simulink model "B1_quadcopter_model"  (R2021b)
settings: Solver=VariableStepAuto  StartTime=0.0  StopTime=10  RelTol=1e-3
values from neighbouring files (symbols this model uses):
  K_act = 50    [A10_simple_plant.m]    (also in A11_setup_script_pprz.m = 20; A1_setup_script.m = 20)
  K_act_inner = K_act*eye(4)    [A11_setup_script_pprz.m]    (also in A1_setup_script.m)
  K_u_d = 2.5    [A11_setup_script_pprz.m]    (also in A1_setup_script.m = 7)
  K_v_d = 2.5    [A11_setup_script_pprz.m]    (also in A1_setup_script.m = 7)
  K_w_d = 2.5    [A11_setup_script_pprz.m]    (also in A1_setup_script.m = 7)
  max_motor_rate = 30000    [A11_setup_script_pprz.m]    (also in A1_setup_script.m)
  max_omega_motor = 11000    [A11_setup_script_pprz.m]    (also in A1_setup_script.m)
  omega_c_motors = 50    [A11_setup_script_pprz.m]    (also in A1_setup_script.m)
  sampling_time = 1/frequency    (= 0.002)    [A11_setup_script_pprz.m]    (also in A12_sim_multi_run.m; A1_setup_script.m; A6_slow_actuator.m)
undefined symbols (not defined in the file or in its folder): K_ec_d_p, K_ec_d_q, K_ec_d_r, K_ec_dd_p, K_ec_dd_q, K_ec_dd_r, K_ec_p, K_ec_q, K_ec_r, K_p, K_p_d, K_p_dd, K_q, K_q_d, K_q_dd, K_r, K_r_d, K_r_dd
libraries: dspinverses x11, simulink_extras x6, sim3dlib x1, uavsim3dlib x1, vrlib x1, aerolibutil x1, sharedutil x1, aerolibbdyn x1, aerolibatmos2 x1
(part 2 of 3)

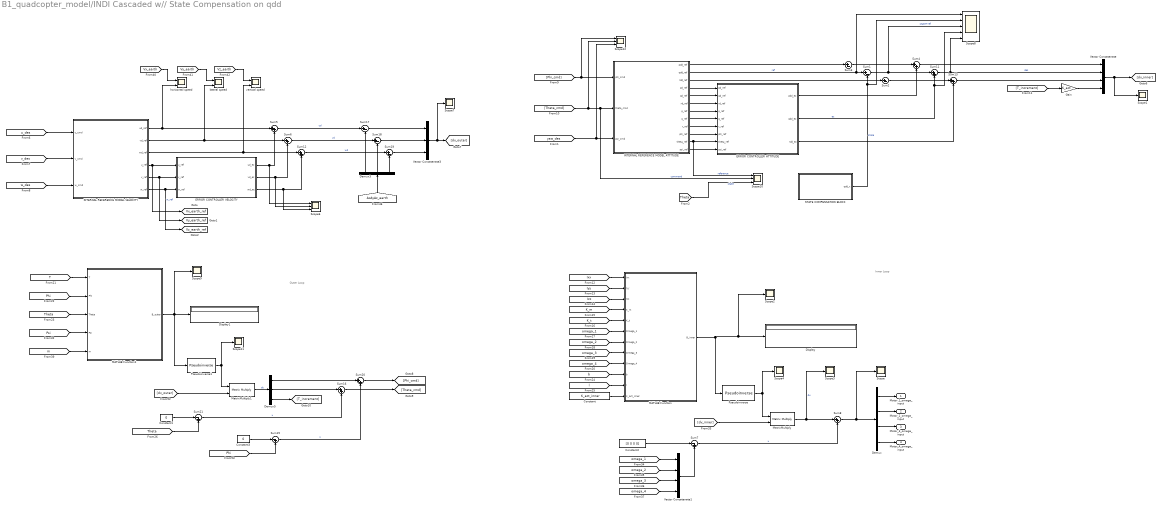
== system B1_quadcopter_model/INDI Cascaded w// State Compensation on qdd ==
  note: Outer Loop
  note: Inner Loop
  Constant : Constant  Value=K_act_inner
  Constant1 : Constant  Value=0
  Constant2 : Constant  Value=[0 0 0 0]
  Constant3 : Constant  Value=0
  Demux : Demux
  Demux3 : Demux  Outputs=3
  Demux5 : Demux  Outputs=3
  Display : Display
  Display1 : Display
  ERROR CONTROLLER ATTITUDE : Subsystem
  ERROR CONTROLLER VELOCITY : Subsystem
  Gain : Gain  Gain=K_act
  INTERNAL REFERENCE MODEL ATTITUDE : Subsystem
  INTERNAL REFERENCE MODEL VELOCITY : Subsystem
  MATLAB Function : MATLAB Function  TreatAsAtomicUnit=on
  MATLAB Function1 : MATLAB Function  TreatAsAtomicUnit=on
  MatrixMultiply : Product  Multiplication=Matrix(*)
  MatrixMultiply1 : Product  Multiplication=Matrix(*)
  Pseudoinverse : dspinverses/Pseudoinverse  wanterr=off  SimulateUsing=Interpreted execution
      settings: SourceProductBaseCode=DS
  Pseudoinverse1 : dspinverses/Pseudoinverse  wanterr=off  SimulateUsing=Interpreted execution
      settings: SourceProductBaseCode=DS
  STATE COMPENSATION BLOCK : Subsystem
  Scope{,1..4,7,9,11} (8 alike) : Scope
  Scope10 : Scope  NumInputPorts=3
  Scope12 : Scope  NumInputPorts=3
  Scope6 : Scope  NumInputPorts=3
  Scope8 : Scope  NumInputPorts=5
  Sum{1..3,17..19} (6 alike) : Sum  Inputs=|+-
  Sum{4..6,8,11..13,16,20} (9 alike) : Sum  Inputs=|++
  Sum15 : Sum  Inputs=|-+
  Sum21 : Sum  Inputs=|-+
  Sum7 : Sum  Inputs=|-+
  Vector Concatenate : Concatenate  NumInputs=4
  Vector Concatenate1 : Concatenate  NumInputs=4
  Vector Concatenate3 : Concatenate  NumInputs=3
  horizontal speed : Scope  NumInputPorts=2
  lateral speed : Scope  NumInputPorts=2
  vertical speed : Scope  NumInputPorts=2
  Motor_1_omega_input : Outport
  Motor_2_omega_input : Outport  Port=2
  Motor_3_omega_input : Outport  Port=3
  Motor_4_omega_input : Outport  Port=4
  tag scope: Vx_earth_ref=global, Vy_earth_ref=global, Vz_earth_ref=global
  wires:
  ERROR CONTROLLER VELOCITY/1(ud_ec) -> Sum5/2, Scope6/1
  ERROR CONTROLLER VELOCITY/3(wd_ec) -> Sum12/2, Scope6/3
  INTERNAL REFERENCE MODEL VELOCITY/3(wd_ref) -> vertical speed/2, Sum12/1
  INTERNAL REFERENCE MODEL VELOCITY/2(vd_ref) -> lateral speed/2, Sum6/1
  INTERNAL REFERENCE MODEL VELOCITY/5(v_ref) -> [Vy_earth_ref], ERROR CONTROLLER VELOCITY/2(v_ref)
  INTERNAL REFERENCE MODEL VELOCITY/6(w_ref) -> [Vz_earth_ref], ERROR CONTROLLER VELOCITY/3(w_ref)  "w_ref"
  INTERNAL REFERENCE MODEL VELOCITY/1(ud_ref) -> horizontal speed/2, Sum5/1
  ERROR CONTROLLER VELOCITY/2(vd_ec) -> Sum6/2, Scope6/2
  INTERNAL REFERENCE MODEL VELOCITY/4(u_ref) -> [Vx_earth_ref], ERROR CONTROLLER VELOCITY/1(u_ref)
  [u_des] -> INTERNAL REFERENCE MODEL VELOCITY/1(u_cmd)
  [v_des] -> INTERNAL REFERENCE MODEL VELOCITY/2(v_cmd)
  [w_des] -> INTERNAL REFERENCE MODEL VELOCITY/3(w_cmd)
  [Phi_cmd] -> Scope12/1, INTERNAL REFERENCE MODEL ATTITUDE/1(phi_cmd)
  [Theta_cmd] -> Scope12/2, Scope10/2, INTERNAL REFERENCE MODEL ATTITUDE/2(theta_cmd)  "command"
  [yaw_des] -> INTERNAL REFERENCE MODEL ATTITUDE/3(psi_cmd), Scope12/3
  Vector Concatenate/1 -> Scope1/1, [dv_inner]
  MATLAB Function/1(B_inner) -> Scope2/1, Display/1, Pseudoinverse/1
  Pseudoinverse/1 -> MatrixMultiply/1, Scope4/1
  MatrixMultiply/1 -> Scope3/1, Sum8/1  "du"
  [omega_1] -> Vector Concatenate1/1
  [omega_2] -> Vector Concatenate1/2
  [omega_3] -> Vector Concatenate1/3
  [omega_4] -> Vector Concatenate1/4
  Vector Concatenate1/1 -> Sum7/2
  Constant2/1 -> Sum7/1
  Sum7/1 -> Sum8/2  "u"
  Sum8/1 -> Scope/1, Demux/1
  Demux/1 -> Motor_1_omega_input/1
  Demux/2 -> Motor_2_omega_input/1
  Demux/3 -> Motor_3_omega_input/1
  Demux/4 -> Motor_4_omega_input/1
  Sum4/1 -> Vector Concatenate/1
  Sum11/1 -> Scope8/5, Vector Concatenate/2  "des"
  Sum13/1 -> Vector Concatenate/3
  [dv_inner] -> MatrixMultiply/2
  [T_increment] -> Gain/1
  Sum12/1 -> Sum19/1  "wd"
  Sum6/1 -> Sum18/1  "vd"
  Sum5/1 -> Sum17/1  "ud"
  Vector Concatenate3/1 -> Scope7/1, [dv_outer]
  [Vz_earth] -> vertical speed/1
  [Vy_earth] -> lateral speed/1
  [Vx_earth] -> horizontal speed/1
  Sum19/1 -> Vector Concatenate3/3
  Sum18/1 -> Vector Concatenate3/2
  Sum17/1 -> Vector Concatenate3/1
  [AxAyAz_earth] -> Demux3/1
  Demux3/3 -> Sum19/2
  Demux3/2 -> Sum18/2
  Demux3/1 -> Sum17/2
  [K_m] -> MATLAB Function/4(K_m)
  [Izz] -> MATLAB Function/3(Izz)
  [Iyy] -> MATLAB Function/2(Iyy)
  [Ixx] -> MATLAB Function/1(Ixx)
  [omega_3] -> MATLAB Function/8(Omega_3)
  [omega_1] -> MATLAB Function/6(Omega_1)
  [omega_4] -> MATLAB Function/9(Omega_4)
  [K_t] -> MATLAB Function/5(K_t)
  [b] -> MATLAB Function/10(b)
  [l] -> MATLAB Function/11(l)
  [omega_2] -> MATLAB Function/7(Omega_2)
  Pseudoinverse1/1 -> Scope11/1, MatrixMultiply1/1
  Sum20/1 -> [Phi_cmd]
  Demux5/1 -> Sum20/1
  [Phi] -> MATLAB Function1/2(Phi)
  Demux5/2 -> Sum16/1
  MatrixMultiply1/1 -> Demux5/1  "du"
  Sum21/1 -> Sum16/2  "u"
  [Theta] -> Sum21/2
  [m] -> MATLAB Function1/5(m)
  [T] -> MATLAB Function1/1(T)
  [dv_outer] -> MatrixMultiply1/2
  Constant1/1 -> Sum21/1
  [Phi] -> Sum15/2
  Sum16/1 -> [Theta_cmd]
  [Psi] -> MATLAB Function1/4(Psi)
  [Theta] -> MATLAB Function1/3(Theta)
  Demux5/3 -> [T_increment]
  Sum15/1 -> Sum20/2  "u"
  MATLAB Function1/1(B_outer) -> Pseudoinverse1/1, Scope9/1, Display1/1
  Constant3/1 -> Sum15/1
  INTERNAL REFERENCE MODEL ATTITUDE/4(pd_ref) -> ERROR CONTROLLER ATTITUDE/1(pd_ref)
  INTERNAL REFERENCE MODEL ATTITUDE/5(qd_ref) -> ERROR CONTROLLER ATTITUDE/2(qd_ref)
  INTERNAL REFERENCE MODEL ATTITUDE/6(rd_ref) -> ERROR CONTROLLER ATTITUDE/3(rd_ref)
  INTERNAL REFERENCE MODEL ATTITUDE/7(p_ref) -> ERROR CONTROLLER ATTITUDE/4(p_ref)
  INTERNAL REFERENCE MODEL ATTITUDE/8(q_ref) -> ERROR CONTROLLER ATTITUDE/5(q_ref)
  INTERNAL REFERENCE MODEL ATTITUDE/9(r_ref) -> ERROR CONTROLLER ATTITUDE/6(r_ref)
  INTERNAL REFERENCE MODEL ATTITUDE/10(phi_ref) -> ERROR CONTROLLER ATTITUDE/7(phi_ref)
  INTERNAL REFERENCE MODEL ATTITUDE/11(theta_ref) -> Scope10/1, ERROR CONTROLLER ATTITUDE/8(theta_ref)  "reference"
  INTERNAL REFERENCE MODEL ATTITUDE/12(psi_ref) -> ERROR CONTROLLER ATTITUDE/9(psi_ref)
  ERROR CONTROLLER ATTITUDE/1(pdd_ec) -> Sum4/2
  ERROR CONTROLLER ATTITUDE/2(qdd_ec) -> Scope8/4, Sum11/2  "ec"
  ERROR CONTROLLER ATTITUDE/3(rdd_ec) -> Sum13/2
  Constant/1 -> MATLAB Function/12(K_act_inner)
  Gain/1 -> Vector Concatenate/4
  Sum2/1 -> Sum13/1
  Sum1/1 -> Scope8/3, Sum11/1  "state+ref"
  Sum3/1 -> Sum4/1
  INTERNAL REFERENCE MODEL ATTITUDE/1(pdd_ref) -> Sum3/1
  INTERNAL REFERENCE MODEL ATTITUDE/2(qdd_ref) -> Scope8/1, Sum1/1  "ref"
  INTERNAL REFERENCE MODEL ATTITUDE/3(rdd_ref) -> Sum2/1
  STATE COMPENSATION BLOCK/1(qdd_x) -> Sum1/2, Scope8/2  "state"
  [Theta] -> Scope10/3  "state"

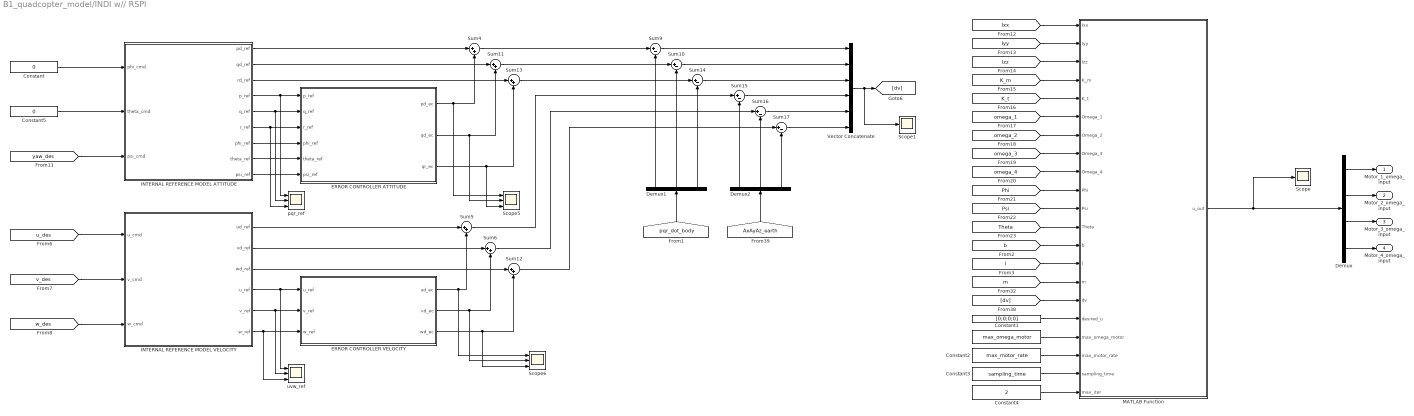
== system B1_quadcopter_model/INDI w// RSPI ==
  " " : Constant  Value=[0;0;0;0]
  Constant : Constant  Value=0
  Constant1 : Constant  Value=max_omega_motor
  Constant2 : Constant  Value=max_motor_rate
  Constant3 : Constant  Value=sampling_time
  Constant4 : Constant  Value=2
  Constant5 : Constant  Value=0
  Demux : Demux
  Demux1 : Demux  Outputs=3
  Demux2 : Demux  Outputs=3
  ERROR CONTROLLER ATTITUDE : Subsystem
  ERROR CONTROLLER VELOCITY : Subsystem
  INTERNAL REFERENCE MODEL ATTITUDE : Subsystem
  INTERNAL REFERENCE MODEL VELOCITY : Subsystem
  MATLAB Function : MATLAB Function  TreatAsAtomicUnit=on
  Scope : Scope
  Scope1 : Scope
  Scope5 : Scope  NumInputPorts=3
  Scope6 : Scope  NumInputPorts=3
  Sum{9..10,14..17} (6 alike) : Sum  Inputs=|+-
  Sum{4..6,11..13} (6 alike) : Sum  Inputs=|++
  Vector Concatenate : Concatenate  NumInputs=6
  pqr_ref : Scope  NumInputPorts=3
  uvw_ref : Scope  NumInputPorts=3
  Motor_1_omega_input : Outport
  Motor_2_omega_input : Outport  Port=2
  Motor_3_omega_input : Outport  Port=3
  Motor_4_omega_input : Outport  Port=4
  wires:
  [Ixx] -> MATLAB Function/1(Ixx)
  [Iyy] -> MATLAB Function/2(Iyy)
  [Izz] -> MATLAB Function/3(Izz)
  [K_m] -> MATLAB Function/4(K_m)
  [K_t] -> MATLAB Function/5(K_t)
  [omega_1] -> MATLAB Function/6(Omega_1)
  [omega_2] -> MATLAB Function/7(Omega_2)
  [omega_3] -> MATLAB Function/8(Omega_3)
  [omega_4] -> MATLAB Function/9(Omega_4)
  [Phi] -> MATLAB Function/10(Phi)
  [Psi] -> MATLAB Function/11(Psi)
  [Theta] -> MATLAB Function/12(Theta)
  [m] -> MATLAB Function/15(m)
  Demux/1 -> Motor_1_omega_input/1
  Demux/2 -> Motor_2_omega_input/1
  Demux/3 -> Motor_3_omega_input/1
  Demux/4 -> Motor_4_omega_input/1
  [dv] -> MATLAB Function/16(dv)
  " "/1 -> MATLAB Function/17(desired_u)
  Constant1/1 -> MATLAB Function/18(max_omega_motor)
  Constant2/1 -> MATLAB Function/19(max_motor_rate)
  Constant3/1 -> MATLAB Function/20(sampling_time)
  MATLAB Function/1(u_out) -> Scope/1, Demux/1
  Constant4/1 -> MATLAB Function/21(max_iter)
  Constant/1 -> INTERNAL REFERENCE MODEL ATTITUDE/1(phi_cmd)
  Constant5/1 -> INTERNAL REFERENCE MODEL ATTITUDE/2(theta_cmd)
  INTERNAL REFERENCE MODEL VELOCITY/5(v_ref) -> ERROR CONTROLLER VELOCITY/2(v_ref), uvw_ref/2
  INTERNAL REFERENCE MODEL ATTITUDE/6(r_ref) -> ERROR CONTROLLER ATTITUDE/3(r_ref), pqr_ref/3
  Demux1/3 -> Sum14/2
  [u_des] -> INTERNAL REFERENCE MODEL VELOCITY/1(u_cmd)
  Sum9/1 -> Vector Concatenate/1
  ERROR CONTROLLER VELOCITY/1(ud_ec) -> Scope6/1, Sum5/2
  [yaw_des] -> INTERNAL REFERENCE MODEL ATTITUDE/3(psi_cmd)
  Vector Concatenate/1 -> Scope1/1, [dv]
  INTERNAL REFERENCE MODEL ATTITUDE/3(rd_ref) -> Sum13/1
  Demux1/1 -> Sum9/2
  INTERNAL REFERENCE MODEL ATTITUDE/5(q_ref) -> ERROR CONTROLLER ATTITUDE/2(q_ref), pqr_ref/2
  Demux2/3 -> Sum17/2
  Sum16/1 -> Vector Concatenate/5
  [pqr_dot_body] -> Demux1/1
  [AxAyAz_earth] -> Demux2/1
  Sum12/1 -> Sum17/1
  Sum10/1 -> Vector Concatenate/2
  Sum14/1 -> Vector Concatenate/3
  ERROR CONTROLLER ATTITUDE/2(qd_ec) -> Scope5/2, Sum11/2
  Demux2/2 -> Sum16/2
  ERROR CONTROLLER ATTITUDE/1(pd_ec) -> Scope5/1, Sum4/2
  Sum15/1 -> Vector Concatenate/4
  Sum17/1 -> Vector Concatenate/6
  ERROR CONTROLLER VELOCITY/3(wd_ec) -> Scope6/3, Sum12/2
  Sum11/1 -> Sum10/1
  INTERNAL REFERENCE MODEL VELOCITY/4(u_ref) -> uvw_ref/1, ERROR CONTROLLER VELOCITY/1(u_ref)
  Sum13/1 -> Sum14/1
  Sum6/1 -> Sum16/1
  INTERNAL REFERENCE MODEL VELOCITY/6(w_ref) -> ERROR CONTROLLER VELOCITY/3(w_ref), uvw_ref/3
  [v_des] -> INTERNAL REFERENCE MODEL VELOCITY/2(v_cmd)
  Demux1/2 -> Sum10/2
  ERROR CONTROLLER VELOCITY/2(vd_ec) -> Scope6/2, Sum6/2
  INTERNAL REFERENCE MODEL VELOCITY/1(ud_ref) -> Sum5/1
  [w_des] -> INTERNAL REFERENCE MODEL VELOCITY/3(w_cmd)
  Sum5/1 -> Sum15/1
  INTERNAL REFERENCE MODEL VELOCITY/3(wd_ref) -> Sum12/1
  Demux2/1 -> Sum15/2
  INTERNAL REFERENCE MODEL ATTITUDE/7(phi_ref) -> ERROR CONTROLLER ATTITUDE/4(phi_ref)
  INTERNAL REFERENCE MODEL ATTITUDE/8(theta_ref) -> ERROR CONTROLLER ATTITUDE/5(theta_ref)
  INTERNAL REFERENCE MODEL ATTITUDE/1(pd_ref) -> Sum4/1
  INTERNAL REFERENCE MODEL VELOCITY/2(vd_ref) -> Sum6/1
  Sum4/1 -> Sum9/1
  INTERNAL REFERENCE MODEL ATTITUDE/4(p_ref) -> pqr_ref/1, ERROR CONTROLLER ATTITUDE/1(p_ref)
  INTERNAL REFERENCE MODEL ATTITUDE/9(psi_ref) -> ERROR CONTROLLER ATTITUDE/6(psi_ref)
  INTERNAL REFERENCE MODEL ATTITUDE/2(qd_ref) -> Sum11/1
  ERROR CONTROLLER ATTITUDE/3(qr_ec) -> Scope5/3, Sum13/2
  [b] -> MATLAB Function/13(b)
  [l] -> MATLAB Function/14(l)

== system B1_quadcopter_model/Quadcopter Characteristics ==
  Gravity : Constant  Value=9.80665
  Moment Gain : Constant  Value=6.68*10^-9
  Plate Distance from CG : Constant  Value=0.1
  Plate Radius (cm) : Constant  Value=0.5
  Quad Inertia Ixx [kg*m^2] : Constant  Value=0.0012458
  Quad Inertia Iyy [kg*m^2] : Constant  Value=0.001500
  Quad Inertia Izz [kg*m^2] : Constant  Value=0.0001500
  Quad Mass [kg] : Constant  Value=0.4
  Thrust Gain : Constant  Value=6.557*10^-8
  lx1 : Constant  Value=0.095
  lx2 : Constant  Value=0.08
  mod scale : Constant
  tag scope: Ixx=global, Iyy=global, Izz=global, K_m=global, K_t=global, b=global, g=global, l=global, l_plate=global, m=global, mod_scale=global, r_plate=global
  wires:
  Quad Inertia Ixx [kg*m^2]/1 -> [Ixx]
  Quad Inertia Iyy [kg*m^2]/1 -> [Iyy]
  Quad Inertia Izz [kg*m^2]/1 -> [Izz]
  Quad Mass [kg]/1 -> [m]
  Thrust Gain/1 -> [K_t]
  Moment Gain/1 -> [K_m]
  lx1/1 -> [b]
  lx2/1 -> [l]
  Plate Radius (cm)/1 -> [r_plate]
  Plate Distance from CG/1 -> [l_plate]
  Gravity/1 -> [g]
  mod scale/1 -> [mod_scale]

== system B1_quadcopter_model/Control Panel Block/Disturbance Block ==
  Step : Step  Time=2  After=3  SampleTime=0
  Step1 : Step  Time=7  After=-3  SampleTime=0
  Sum : Sum  Inputs=|++
  Total Disturbance : Outport
  wires:
  Step/1 -> Sum/1
  Sum/1 -> Total Disturbance/1
  Step1/1 -> Sum/2

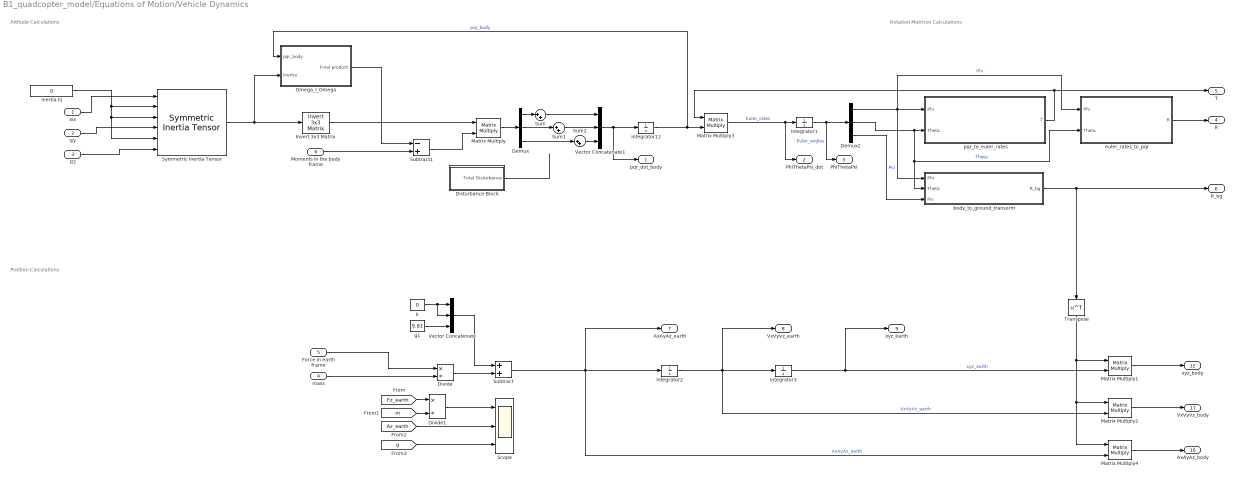
== system B1_quadcopter_model/Equations of Motion/Vehicle Dynamics ==
  note: Attitude Calculations
  note: Rotation Matrices Calculations
  note: Position Calculations
  Ixx : Inport
  Iyy : Inport  Port=2
  Izz : Inport  Port=3
  mass : Inport  Port=4
  Force in earth frame : Inport  Port=5
  Moments in the body frame : Inport  Port=6
  Demux : Demux  Outputs=3
  Demux2 : Demux  Outputs=3
  Disturbance Block : Subsystem
  Divide : Product  Inputs=*/
  Divide1 : Product  Inputs=*/
  Inertia Iij : Constant  Value=0
  Integrator{1..3,12} (4 alike) : Integrator
  Invert 3x3 Matrix : aerolibutil/Invert  3x3 Matrix
  Matrix Multiply{,1..4} (5 alike) : Product  Multiplication=Matrix(*)
  Omega_I_Omega : Subsystem
  Scope : Scope  NumInputPorts=3
  Subtract : Sum
  Subtract1 : Sum  Inputs=-+
  Sum : Sum  Inputs=|++
  Sum1 : Sum  Inputs=|++
  Sum2 : Sum  Inputs=|++
  Symmetric Inertia Tensor : aerolibbdyn/Symmetric Inertia Tensor
      settings: SourceProductBaseCode=AE
  Transpose : Math  Operator=transpose  SaturateOnIntegerOverflow=on
  Vector Concatenate : Concatenate  NumInputs=3
  Vector Concatenate1 : Concatenate  NumInputs=3
  body_to_ground_transorm : MATLAB Function  Description=|  TreatAsAtomicUnit=on
      | This function computes the rotational matrix to pass from the body frame to the world frame. 
      | Takes as inpout the euler angles.
  euler_rates_to_pqr : MATLAB Function  TreatAsAtomicUnit=on
  g1 : Constant  Value=9.81  VectorParams1D=off
  k : Constant  Value=0  VectorParams1D=off
  pqr_to_euler_rates : MATLAB Function  TreatAsAtomicUnit=on
  pqr_dot_body : Outport
  PhiThetaPsi_dot : Outport  Port=2
  PhiThetaPsi : Outport  Port=3
  R : Outport  Port=4
  T : Outport  Port=5
  R_bg : Outport  Port=6
  AxAyAz_earth : Outport  Port=7
  VxVyVz_earth : Outport  Port=8
  xyz_earth : Outport  Port=9
  AxAyAz_body : Outport  Port=10
  VxVyVz_body : Outport  Port=11
  xyz_body : Outport  Port=12
  wires:
  Transpose/1 -> Matrix Multiply1/1, Matrix Multiply2/1, Matrix Multiply4/1
  Matrix Multiply2/1 -> VxVyVz_body/1
  Matrix Multiply1/1 -> xyz_body/1
  Subtract/1 -> Integrator2/1, Matrix Multiply4/2, AxAyAz_earth/1  "AxAyAz_earth"
  Matrix Multiply4/1 -> AxAyAz_body/1
  body_to_ground_transorm/1(R_bg) -> Transpose/1, R_bg/1
  Integrator2/1 -> Matrix Multiply2/2, VxVyVz_earth/1, Integrator3/1  "VxVyVz_earth"
  Force in earth frame/1 -> Divide/1
  Demux2/3 -> body_to_ground_transorm/3(Psi)  "Psi"
  Demux2/2 -> euler_rates_to_pqr/2(Theta), body_to_ground_transorm/2(Theta), pqr_to_euler_rates/2(Theta)  "Theta"
  euler_rates_to_pqr/1(R) -> R/1
  pqr_to_euler_rates/1(T) -> Matrix Multiply3/1, T/1
  Matrix Multiply/1 -> Demux/1
  Integrator12/1 -> Matrix Multiply3/2, Omega_I_Omega/1(pqr_body)  "pqr_body"
  Integrator3/1 -> Matrix Multiply1/2, xyz_earth/1  "xyz_earth"
  Ixx/1 -> Symmetric Inertia Tensor/1
  k/1 -> Vector Concatenate/2, Vector Concatenate/1
  Vector Concatenate/1 -> Subtract/1
  Integrator1/1 -> PhiThetaPsi/1, Demux2/1  "Euler_angles"
  g1/1 -> Vector Concatenate/3
  Moments in the body frame/1 -> Subtract1/2
  Demux2/1 -> euler_rates_to_pqr/1(Phi), pqr_to_euler_rates/1(Phi), body_to_ground_transorm/1(Phi)  "Phi"
  Vector Concatenate1/1 -> Integrator12/1, pqr_dot_body/1
  Matrix Multiply3/1 -> PhiThetaPsi_dot/1, Integrator1/1  "Euler_rates"
  mass/1 -> Divide/2
  Omega_I_Omega/1(Final product) -> Subtract1/1
  Subtract1/1 -> Matrix Multiply/2
  Invert 3x3 Matrix/1 -> Matrix Multiply/1
  Inertia Iij/1 -> Symmetric Inertia Tensor/5, Symmetric Inertia Tensor/3, Symmetric Inertia Tensor/2
  Divide/1 -> Subtract/2
  Symmetric Inertia Tensor/1 -> Invert 3x3 Matrix/1, Omega_I_Omega/2(Inertia)
  Iyy/1 -> Symmetric Inertia Tensor/4
  Izz/1 -> Symmetric Inertia Tensor/6
  [Fz_earth] -> Divide1/1
  [m] -> Divide1/2
  Divide1/1 -> Scope/1
  [Az_earth] -> Scope/2
  [g] -> Scope/3
  Demux/1 -> Sum/1
  Sum/1 -> Vector Concatenate1/1
  Sum2/1 -> Vector Concatenate1/3
  Sum1/1 -> Vector Concatenate1/2
  Demux/2 -> Sum1/1
  Demux/3 -> Sum2/1
  Disturbance Block/1(Total Disturbance) -> ?

== system B1_quadcopter_model/Force and Moment Calculation/Forces and Moments due to Aerodynamic Forces ==
  z_earth : Inport
  R_bg : Inport  Port=2
  Aerodynamic Forces Calculator : MATLAB Function  TreatAsAtomicUnit=on
  Constant : Constant  Value=0
  Gain : Gain  Gain=-1
  ISA Atmosphere Model : aerolibatmos2/ISA Atmosphere Model  custom=off  g=9.80665  gamma=1.4  R=287.0531  L=0.0065  h_trop=11000  h_strat=20000  rho0=1.225  P0=101325  T0=288.15  h0=0
  Matrix Multiply1 : Product  Multiplication=Matrix(*)
  Radians to Degrees : simulink_extras/Transformations/Radians to Degrees
  Radians to Degrees1 : simulink_extras/Transformations/Radians to Degrees
  Scope : Scope  NumInputPorts=6
  Scope1 : Scope  NumInputPorts=2
  Scope2 : Scope  NumInputPorts=2
  Scope3 : Scope  NumInputPorts=2
  Scope4 : Scope
  Switch : Switch  Criteria=u2 > Threshold
  Terminator : Terminator
  Terminator1 : Terminator
  Terminator2 : Terminator
  Vector Concatenate : Concatenate  NumInputs=3
  Vector Concatenate1 : Concatenate  NumInputs=3
  F_aero : Outport
  M_aero : Outport  Port=2
  tag scope: alpha=global, beta=global, rho=global
  wires:
  ISA Atmosphere Model/2 -> Terminator1/1
  ISA Atmosphere Model/1 -> Terminator/1
  ISA Atmosphere Model/3 -> Terminator2/1
  z_earth/1 -> Gain/1
  ISA Atmosphere Model/4 -> Scope4/1, [rho]
  Aerodynamic Forces Calculator/3(Fz_body) -> Scope/3, Vector Concatenate/3  "Fz_body"
  Aerodynamic Forces Calculator/2(Fy_body) -> Scope/2, Vector Concatenate/2  "Fy_body"
  Matrix Multiply1/1 -> F_aero/1
  R_bg/1 -> Matrix Multiply1/1
  Aerodynamic Forces Calculator/1(Fx_body) -> Scope/1, Vector Concatenate/1  "Fx_body"
  Vector Concatenate/1 -> Matrix Multiply1/2
  Aerodynamic Forces Calculator/4(L_aero) -> Scope/4, Vector Concatenate1/1  "Mx"
  Aerodynamic Forces Calculator/5(M_aero) -> Scope/5, Vector Concatenate1/2  "My"
  Aerodynamic Forces Calculator/6(N_aero) -> Scope/6, Vector Concatenate1/3  "Mz"
  Vector Concatenate1/1 -> M_aero/1
  [Vx_body] -> Aerodynamic Forces Calculator/1(xd_body)
  [Vy_body] -> Aerodynamic Forces Calculator/2(yd_body)
  [Vz_body] -> Aerodynamic Forces Calculator/3(zd_body)
  [rho] -> Aerodynamic Forces Calculator/4(rho)
  [r_plate] -> Aerodynamic Forces Calculator/5(r_plate)
  [l_plate] -> Aerodynamic Forces Calculator/6(l_plate)
  Gain/1 -> Switch/2, Switch/1
  Constant/1 -> Switch/3
  Switch/1 -> ISA Atmosphere Model/1
  Aerodynamic Forces Calculator/7(Cl) -> Scope1/1  "Cl"
  Aerodynamic Forces Calculator/8(Cd) -> Scope1/2  "Cd"
  Aerodynamic Forces Calculator/9(L) -> Scope2/1  "L"
  Aerodynamic Forces Calculator/10(D) -> Scope2/2  "D"
  Aerodynamic Forces Calculator/11(alpha) -> [alpha], Radians to Degrees/1  "alpha"
  Aerodynamic Forces Calculator/12(beta) -> [beta], Radians to Degrees1/1  "beta"
  Radians to Degrees/1 -> Scope3/1
  Radians to Degrees1/1 -> Scope3/2
  [mod_scale] -> Aerodynamic Forces Calculator/7(mod_scale)

== system B1_quadcopter_model/INDI Block/ERROR CONTROLLER ATTITUDE ==
  p_ref : Inport
  q_ref : Inport  Port=2
  r_ref : Inport  Port=3
  phi_ref : Inport  Port=4
  theta_ref : Inport  Port=5
  psi_ref : Inport  Port=6
  Demux5 : Demux  Outputs=3
  Gain{,1..5} (6 alike) : Gain
  Sum{,1,3..4,6..7} (6 alike) : Sum  Inputs=|+-
  Sum2 : Sum  Inputs=|++
  Sum5 : Sum  Inputs=|++
  Sum8 : Sum  Inputs=|++
  pd_ec : Outport
  qd_ec : Outport  Port=2
  qr_ec : Outport  Port=3
  wires:
  p_ref/1 -> Sum/1
  phi_ref/1 -> Sum1/1
  Sum/1 -> Gain/1
  Sum1/1 -> Gain1/1
  Gain/1 -> Sum2/1
  Gain1/1 -> Sum2/2
  Sum2/1 -> pd_ec/1
  Gain2/1 -> Sum5/1
  Sum3/1 -> Gain2/1
  Gain3/1 -> Sum5/2
  theta_ref/1 -> Sum4/1
  q_ref/1 -> Sum3/1
  Sum5/1 -> qd_ec/1
  Sum4/1 -> Gain3/1
  Gain4/1 -> Sum8/1
  Sum6/1 -> Gain4/1
  Gain5/1 -> Sum8/2
  psi_ref/1 -> Sum7/1
  r_ref/1 -> Sum6/1
  Sum8/1 -> qr_ec/1
  Sum7/1 -> Gain5/1
  [Phi] -> Sum1/2
  [Theta] -> Sum4/2
  [Psi] -> Sum7/2
  Demux5/1 -> Sum/2
  Demux5/2 -> Sum3/2
  Demux5/3 -> Sum6/2
  [PhiThetaPsi_dot] -> Demux5/1

== system B1_quadcopter_model/INDI Block/ERROR CONTROLLER VELOCITY ==
  u_ref : Inport
  v_ref : Inport  Port=2
  w_ref : Inport  Port=3
  Gain : Gain
  Gain2 : Gain
  Gain4 : Gain
  Sum : Sum  Inputs=|+-
  Sum3 : Sum  Inputs=|+-
  Sum6 : Sum  Inputs=|+-
  ud_ec : Outport
  vd_ec : Outport  Port=2
  wd_ec : Outport  Port=3
  wires:
  u_ref/1 -> Sum/1
  Sum/1 -> Gain/1
  Gain/1 -> ud_ec/1
  Sum3/1 -> Gain2/1
  v_ref/1 -> Sum3/1
  Gain2/1 -> vd_ec/1
  Sum6/1 -> Gain4/1
  w_ref/1 -> Sum6/1
  [Vx_earth] -> Sum/2
  [Vz_earth] -> Sum6/2
  [Vy_earth] -> Sum3/2
  Gain4/1 -> wd_ec/1

== system B1_quadcopter_model/INDI Block/INTERNAL REFERENCE MODEL ATTITUDE ==
  phi_cmd : Inport
  theta_cmd : Inport  Port=2
  psi_cmd : Inport  Port=3
  Gain1 : Gain
  Gain10 : Gain  Gain=2
  Gain11 : Gain  Gain=2
  Gain7 : Gain
  Gain8 : Gain  Gain=2
  Gain9 : Gain
  Integrator{,1..5} (6 alike) : Integrator
  Sum{1,11,16,20..22} (6 alike) : Sum  Inputs=|+-
  pd_ref : Outport
  qd_ref : Outport  Port=2
  rd_ref : Outport  Port=3
  p_ref : Outport  Port=4
  q_ref : Outport  Port=5
  r_ref : Outport  Port=6
  phi_ref : Outport  Port=7
  theta_ref : Outport  Port=8
  psi_ref : Outport  Port=9
  wires:
  Integrator1/1 -> Sum11/2, theta_ref/1
  Gain11/1 -> rd_ref/1, Integrator4/1
  Integrator2/1 -> Integrator3/1, p_ref/1, Sum21/2
  Integrator4/1 -> Integrator5/1, r_ref/1, Sum22/2
  Integrator/1 -> Integrator1/1, q_ref/1, Sum16/2
  Gain7/1 -> Sum16/1
  Gain9/1 -> Sum21/1
  Gain1/1 -> Sum22/1
  Gain8/1 -> qd_ref/1, Integrator/1
  Sum21/1 -> Gain10/1
  Sum11/1 -> Gain7/1
  Sum22/1 -> Gain11/1
  Sum16/1 -> Gain8/1
  Integrator3/1 -> phi_ref/1, Sum20/2
  Sum20/1 -> Gain9/1
  Gain10/1 -> pd_ref/1, Integrator2/1
  phi_cmd/1 -> Sum20/1
  theta_cmd/1 -> Sum11/1
  psi_cmd/1 -> Sum1/1
  Integrator5/1 -> Sum1/2, psi_ref/1
  Sum1/1 -> Gain1/1

== system B1_quadcopter_model/INDI Block/INTERNAL REFERENCE MODEL VELOCITY ==
  u_cmd : Inport
  v_cmd : Inport  Port=2
  w_cmd : Inport  Port=3
  Gain1 : Gain  Gain=2
  Gain7 : Gain  Gain=2
  Gain9 : Gain  Gain=2
  Integrator1 : Integrator
  Integrator3 : Integrator
  Integrator5 : Integrator
  Sum1 : Sum  Inputs=|+-
  Sum11 : Sum  Inputs=|+-
  Sum20 : Sum  Inputs=|+-
  ud_ref : Outport
  vd_ref : Outport  Port=2
  wd_ref : Outport  Port=3
  u_ref : Outport  Port=4
  v_ref : Outport  Port=5
  w_ref : Outport  Port=6
  wires:
  Integrator1/1 -> w_ref/1, Sum11/2
  Gain7/1 -> Integrator1/1, wd_ref/1
  Gain9/1 -> ud_ref/1, Integrator3/1
  v_cmd/1 -> Sum1/1
  Sum11/1 -> Gain7/1
  Integrator3/1 -> Sum20/2, u_ref/1
  Sum20/1 -> Gain9/1
  u_cmd/1 -> Sum20/1
  w_cmd/1 -> Sum11/1
  Integrator5/1 -> Sum1/2, v_ref/1
  Gain1/1 -> vd_ref/1, Integrator5/1
  Sum1/1 -> Gain1/1

== system B1_quadcopter_model/INDI Cascaded/ERROR CONTROLLER ATTITUDE ==
  p_ref : Inport
  q_ref : Inport  Port=2
  r_ref : Inport  Port=3
  phi_ref : Inport  Port=4
  theta_ref : Inport  Port=5
  psi_ref : Inport  Port=6
  Demux5 : Demux  Outputs=3
  Gain : Gain  Gain=K_ec_d_p
  Gain1 : Gain  Gain=K_ec_p
  Gain2 : Gain  Gain=K_ec_d_q
  Gain3 : Gain  Gain=K_ec_q
  Gain4 : Gain  Gain=K_ec_d_r
  Gain5 : Gain  Gain=K_ec_r
  Integrator : Integrator
  Scope : Scope  NumInputPorts=2
  Sum{,1,3..4,6..7} (6 alike) : Sum  Inputs=|+-
  Sum2 : Sum  Inputs=|++
  Sum5 : Sum  Inputs=|++
  Sum8 : Sum  Inputs=|++
  pd_ec : Outport
  qd_ec : Outport  Port=2
  qr_ec : Outport  Port=3
  wires:
  p_ref/1 -> Sum/1
  phi_ref/1 -> Sum1/1
  Sum/1 -> Gain/1
  Sum1/1 -> Gain1/1
  Sum2/1 -> pd_ec/1
  Sum3/1 -> Gain2/1
  theta_ref/1 -> Scope/1, Sum4/1
  q_ref/1 -> Sum3/1
  Sum5/1 -> qd_ec/1
  Sum4/1 -> Gain3/1
  Sum6/1 -> Gain4/1
  psi_ref/1 -> Sum7/1
  r_ref/1 -> Sum6/1
  Sum8/1 -> qr_ec/1
  Sum7/1 -> Gain5/1
  [Phi] -> Sum1/2
  [Theta] -> Scope/2, Sum4/2
  [Psi] -> Sum7/2
  Demux5/1 -> Sum/2
  Demux5/2 -> Sum3/2
  Demux5/3 -> Sum6/2
  [pqr_dot_body] -> Integrator/1
  Integrator/1 -> Demux5/1
  Gain2/1 -> Sum5/1
  Gain4/1 -> Sum8/1
  Gain3/1 -> Sum5/2
  Gain1/1 -> Sum2/2
  Gain/1 -> Sum2/1
  Gain5/1 -> Sum8/2

== system B1_quadcopter_model/INDI Cascaded/ERROR CONTROLLER VELOCITY ==
  u_ref : Inport
  v_ref : Inport  Port=2
  w_ref : Inport  Port=3
  Gain{,1..5} (6 alike) : Gain  Gain=5
  Integrator : Integrator
  Integrator1 : Integrator
  Integrator2 : Integrator
  Sum : Sum  Inputs=|+-
  Sum1 : Sum  Inputs=|++
  Sum2 : Sum  Inputs=|++
  Sum3 : Sum  Inputs=|+-
  Sum4 : Sum  Inputs=|++
  Sum6 : Sum  Inputs=|+-
  ud_ec : Outport
  vd_ec : Outport  Port=2
  wd_ec : Outport  Port=3
  wires:
  [Vz_earth] -> Sum6/2
  Gain3/1 -> Sum2/2
  Gain1/1 -> Sum1/2
  Sum1/1 -> ud_ec/1
  Gain2/1 -> Sum2/1
  Integrator2/1 -> Gain5/1
  Sum2/1 -> vd_ec/1
  v_ref/1 -> Sum3/1
  Gain4/1 -> Sum4/1
  Integrator1/1 -> Gain3/1
  Gain/1 -> Sum1/1
  u_ref/1 -> Sum/1
  Sum6/1 -> Integrator2/1, Gain4/1
  [Vy_earth] -> Sum3/2
  w_ref/1 -> Sum6/1
  Sum/1 -> Integrator/1, Gain/1
  Sum4/1 -> wd_ec/1
  Gain5/1 -> Sum4/2
  [Vx_earth] -> Sum/2
  Sum3/1 -> Integrator1/1, Gain2/1
  Integrator/1 -> Gain1/1

== system B1_quadcopter_model/INDI Cascaded/INTERNAL REFERENCE MODEL ATTITUDE ==
  phi_cmd : Inport
  theta_cmd : Inport  Port=2
  psi_cmd : Inport  Port=3
  Gain : Gain  Gain=K_p_d
  Gain1 : Gain  Gain=K_p
  Gain2 : Gain  Gain=K_q
  Gain3 : Gain  Gain=K_r
  Gain4 : Gain  Gain=K_q_d
  Gain5 : Gain  Gain=K_r_d
  Integrator{,1..5} (6 alike) : Integrator
  Subsystem : Subsystem
  Subsystem1 : Subsystem
  Sum{1,11,16,20..22} (6 alike) : Sum  Inputs=|+-
  pd_ref : Outport
  qd_ref : Outport  Port=2
  rd_ref : Outport  Port=3
  p_ref : Outport  Port=4
  q_ref : Outport  Port=5
  r_ref : Outport  Port=6
  phi_ref : Outport  Port=7
  theta_ref : Outport  Port=8
  psi_ref : Outport  Port=9
  wires:
  Integrator1/1 -> Sum11/2, theta_ref/1
  Integrator2/1 -> p_ref/1, Subsystem1/1(p), Sum21/2
  Gain5/1 -> rd_ref/1, Integrator4/1
  Subsystem1/1(dphi) -> Integrator3/1
  Subsystem1/3(dpsi) -> Integrator5/1
  Subsystem1/2(dtheta) -> Integrator1/1
  Subsystem/2(q) -> Sum16/1
  Subsystem/1(p) -> Sum21/1
  Subsystem/3(r) -> Sum22/1
  Gain4/1 -> qd_ref/1, Integrator/1
  Sum11/1 -> Gain2/1
  Integrator3/1 -> phi_ref/1, Sum20/2
  Sum20/1 -> Gain1/1
  Integrator4/1 -> r_ref/1, Subsystem1/3(r), Sum22/2
  Gain/1 -> pd_ref/1, Integrator2/1
  Integrator/1 -> q_ref/1, Subsystem1/2(q), Sum16/2
  phi_cmd/1 -> Sum20/1
  theta_cmd/1 -> Sum11/1
  psi_cmd/1 -> Sum1/1
  Integrator5/1 -> Sum1/2, psi_ref/1
  Sum1/1 -> Gain3/1
  Gain1/1 -> Subsystem/1(dphi)
  Sum21/1 -> Gain/1
  Gain2/1 -> Subsystem/2(dtheta)
  Gain3/1 -> Subsystem/3(dpsi)
  Sum16/1 -> Gain4/1
  Sum22/1 -> Gain5/1

== system B1_quadcopter_model/INDI Cascaded/INTERNAL REFERENCE MODEL VELOCITY ==
  u_cmd : Inport
  v_cmd : Inport  Port=2
  w_cmd : Inport  Port=3
  Gain1 : Gain  Gain=K_w_d
  Gain2 : Gain  Gain=K_v_d
  Gain9 : Gain  Gain=K_u_d
  Integrator1 : Integrator
  Integrator3 : Integrator
  Integrator5 : Integrator
  Sum1 : Sum  Inputs=|+-
  Sum11 : Sum  Inputs=|+-
  Sum20 : Sum  Inputs=|+-
  ud_ref : Outport
  vd_ref : Outport  Port=2
  wd_ref : Outport  Port=3
  u_ref : Outport  Port=4
  v_ref : Outport  Port=5
  w_ref : Outport  Port=6
  wires:
  Integrator1/1 -> w_ref/1, Sum11/2
  Gain1/1 -> Integrator1/1, wd_ref/1
  Gain9/1 -> ud_ref/1, Integrator3/1
  v_cmd/1 -> Sum1/1
  Integrator3/1 -> Sum20/2, u_ref/1
  u_cmd/1 -> Sum20/1
  w_cmd/1 -> Sum11/1
  Integrator5/1 -> Sum1/2, v_ref/1
  Gain2/1 -> vd_ref/1, Integrator5/1
  Sum1/1 -> Gain2/1
  Sum11/1 -> Gain1/1
  Sum20/1 -> Gain9/1

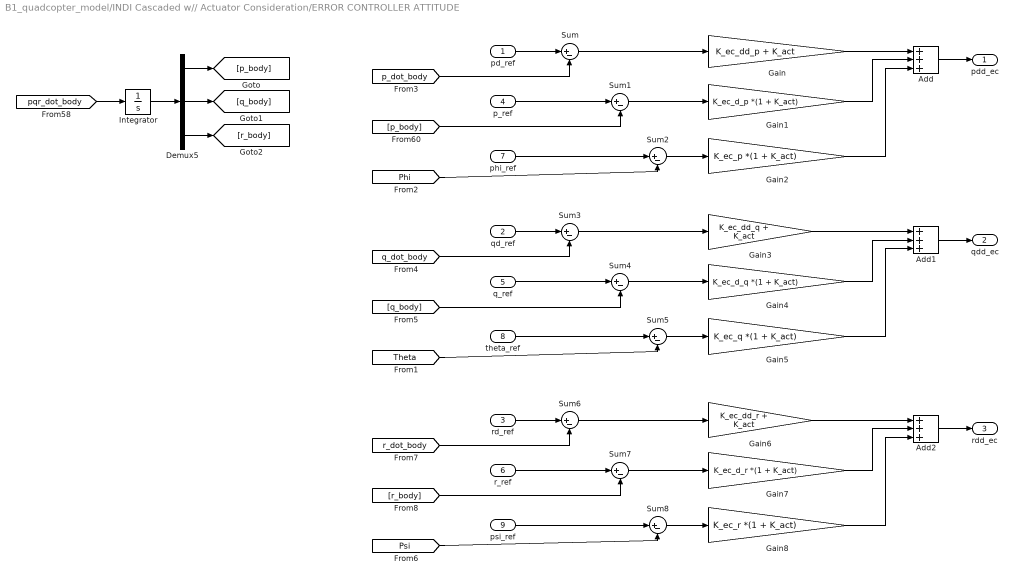
== system B1_quadcopter_model/INDI Cascaded w// Actuator Consideration/ERROR CONTROLLER ATTITUDE ==
  pd_ref : Inport
  qd_ref : Inport  Port=2
  rd_ref : Inport  Port=3
  p_ref : Inport  Port=4
  q_ref : Inport  Port=5
  r_ref : Inport  Port=6
  phi_ref : Inport  Port=7
  theta_ref : Inport  Port=8
  psi_ref : Inport  Port=9
  Add : Sum  Inputs=+++
  Add1 : Sum  Inputs=+++
  Add2 : Sum  Inputs=+++
  Demux5 : Demux  Outputs=3
  Gain : Gain  Gain=K_ec_dd_p + K_act
  Gain1 : Gain  Gain=K_ec_d_p *(1 + K_act)
  Gain2 : Gain  Gain=K_ec_p *(1 + K_act)
  Gain3 : Gain  Gain=K_ec_dd_q + K_act
  Gain4 : Gain  Gain=K_ec_d_q *(1 + K_act)
  Gain5 : Gain  Gain=K_ec_q *(1 + K_act)
  Gain6 : Gain  Gain=K_ec_dd_r + K_act
  Gain7 : Gain  Gain=K_ec_d_r *(1 + K_act)
  Gain8 : Gain  Gain=K_ec_r *(1 + K_act)
  Integrator : Integrator
  Sum{,1..8} (9 alike) : Sum  Inputs=|+-
  pdd_ec : Outport
  qdd_ec : Outport  Port=2
  rdd_ec : Outport  Port=3
  wires:
  pd_ref/1 -> Sum/1
  p_ref/1 -> Sum1/1
  Add/1 -> pdd_ec/1
  [p_body] -> Sum1/2
  [pqr_dot_body] -> Integrator/1
  Integrator/1 -> Demux5/1
  [Phi] -> Sum2/2
  phi_ref/1 -> Sum2/1
  Demux5/2 -> [q_body]
  Demux5/1 -> [p_body]
  Demux5/3 -> [r_body]
  [p_dot_body] -> Sum/2
  Sum/1 -> Gain/1
  Gain/1 -> Add/1
  Sum1/1 -> Gain1/1
  Sum2/1 -> Gain2/1
  Gain1/1 -> Add/2
  Gain2/1 -> Add/3
  Sum4/1 -> Gain4/1
  Sum5/1 -> Gain5/1
  Sum3/1 -> Gain3/1
  [q_dot_body] -> Sum3/2
  Gain4/1 -> Add1/2
  Gain5/1 -> Add1/3
  theta_ref/1 -> Sum5/1
  [Theta] -> Sum5/2
  [q_body] -> Sum4/2
  Gain3/1 -> Add1/1
  q_ref/1 -> Sum4/1
  Add1/1 -> qdd_ec/1
  qd_ref/1 -> Sum3/1
  Sum7/1 -> Gain7/1
  Sum8/1 -> Gain8/1
  Sum6/1 -> Gain6/1
  [r_dot_body] -> Sum6/2
  Gain7/1 -> Add2/2
  Gain8/1 -> Add2/3
  psi_ref/1 -> Sum8/1
  [Psi] -> Sum8/2
  [r_body] -> Sum7/2
  Gain6/1 -> Add2/1
  r_ref/1 -> Sum7/1
  Add2/1 -> rdd_ec/1
  rd_ref/1 -> Sum6/1

== system B1_quadcopter_model/INDI Cascaded w// Actuator Consideration/ERROR CONTROLLER VELOCITY ==
  u_ref : Inport
  v_ref : Inport  Port=2
  w_ref : Inport  Port=3
  Gain{,1..5} (6 alike) : Gain  Gain=5
  Integrator : Integrator
  Integrator1 : Integrator
  Integrator2 : Integrator
  Sum : Sum  Inputs=|+-
  Sum1 : Sum  Inputs=|++
  Sum2 : Sum  Inputs=|++
  Sum3 : Sum  Inputs=|+-
  Sum4 : Sum  Inputs=|++
  Sum6 : Sum  Inputs=|+-
  ud_ec : Outport
  vd_ec : Outport  Port=2
  wd_ec : Outport  Port=3
  wires:
  [Vz_earth] -> Sum6/2
  Gain3/1 -> Sum2/2
  Gain1/1 -> Sum1/2
  Sum1/1 -> ud_ec/1
  Gain2/1 -> Sum2/1
  Integrator2/1 -> Gain5/1
  Sum2/1 -> vd_ec/1
  v_ref/1 -> Sum3/1
  Gain4/1 -> Sum4/1
  Integrator1/1 -> Gain3/1
  Gain/1 -> Sum1/1
  u_ref/1 -> Sum/1
  Sum6/1 -> Integrator2/1, Gain4/1
  [Vy_earth] -> Sum3/2
  w_ref/1 -> Sum6/1
  Sum/1 -> Integrator/1, Gain/1
  Sum4/1 -> wd_ec/1
  Gain5/1 -> Sum4/2
  [Vx_earth] -> Sum/2
  Sum3/1 -> Integrator1/1, Gain2/1
  Integrator/1 -> Gain1/1

== system B1_quadcopter_model/INDI Cascaded w// Actuator Consideration/INTERNAL REFERENCE MODEL ATTITUDE ==
  phi_cmd : Inport
  theta_cmd : Inport  Port=2
  psi_cmd : Inport  Port=3
  Gain1 : Gain  Gain=K_q_dd
  Gain2 : Gain  Gain=K_p_dd
  Gain3 : Gain  Gain=K_r_dd
  Gain4 : Gain  Gain=K_p_d
  Gain5 : Gain  Gain=K_q_d
  Gain6 : Gain  Gain=K_r_d
  Gain7 : Gain  Gain=K_p
  Gain8 : Gain  Gain=K_q
  Gain9 : Gain  Gain=K_r
  Integrator{,1..8} (9 alike) : Integrator
  Subsystem : Subsystem
  Subsystem1 : Subsystem
  Sum{1..4,11,16,20..22} (9 alike) : Sum  Inputs=|+-
  pdd_ref : Outport
  qdd_ref : Outport  Port=2
  rdd_ref : Outport  Port=3
  pd_ref : Outport  Port=4
  qd_ref : Outport  Port=5
  rd_ref : Outport  Port=6
  p_ref : Outport  Port=7
  q_ref : Outport  Port=8
  r_ref : Outport  Port=9
  phi_ref : Outport  Port=10
  theta_ref : Outport  Port=11
  psi_ref : Outport  Port=12
  wires:
  Integrator1/1 -> theta_ref/1, Sum11/2
  Integrator2/1 -> p_ref/1, Subsystem1/1(p), Sum21/2
  Integrator8/1 -> Sum4/2, rd_ref/1, Integrator4/1
  Subsystem1/1(dphi) -> Integrator3/1
  Subsystem1/3(dpsi) -> Integrator5/1
  Subsystem1/2(dtheta) -> Integrator1/1
  Subsystem/2(q) -> Sum16/1
  Subsystem/1(p) -> Sum21/1
  Subsystem/3(r) -> Sum22/1
  Integrator7/1 -> Sum3/2, qd_ref/1, Integrator/1
  Sum21/1 -> Gain4/1
  Sum11/1 -> Gain8/1
  Sum22/1 -> Gain6/1
  Sum16/1 -> Gain5/1
  Integrator3/1 -> phi_ref/1, Sum20/2
  Sum20/1 -> Gain7/1
  Integrator4/1 -> r_ref/1, Subsystem1/3(r), Sum22/2
  Integrator6/1 -> Sum2/2, pd_ref/1, Integrator2/1
  Integrator/1 -> q_ref/1, Subsystem1/2(q), Sum16/2
  phi_cmd/1 -> Sum20/1
  theta_cmd/1 -> Sum11/1
  psi_cmd/1 -> Sum1/1
  Integrator5/1 -> psi_ref/1, Sum1/2
  Sum1/1 -> Gain9/1
  Gain7/1 -> Subsystem/1(dphi)
  Gain8/1 -> Subsystem/2(dtheta)
  Gain9/1 -> Subsystem/3(dpsi)
  Gain4/1 -> Sum2/1
  Gain5/1 -> Sum3/1
  Gain6/1 -> Sum4/1
  Sum2/1 -> Gain2/1
  Sum3/1 -> Gain1/1
  Sum4/1 -> Gain3/1
  Gain2/1 -> pdd_ref/1, Integrator6/1
  Gain1/1 -> qdd_ref/1, Integrator7/1
  Gain3/1 -> rdd_ref/1, Integrator8/1

== system B1_quadcopter_model/INDI Cascaded w// Actuator Consideration/INTERNAL REFERENCE MODEL VELOCITY ==
  u_cmd : Inport
  v_cmd : Inport  Port=2
  w_cmd : Inport  Port=3
  Gain1 : Gain  Gain=2
  Gain7 : Gain  Gain=2
  Gain9 : Gain  Gain=2
  Integrator1 : Integrator
  Integrator3 : Integrator
  Integrator5 : Integrator
  Sum1 : Sum  Inputs=|+-
  Sum11 : Sum  Inputs=|+-
  Sum20 : Sum  Inputs=|+-
  ud_ref : Outport
  vd_ref : Outport  Port=2
  wd_ref : Outport  Port=3
  u_ref : Outport  Port=4
  v_ref : Outport  Port=5
  w_ref : Outport  Port=6
  wires:
  Integrator1/1 -> w_ref/1, Sum11/2
  Gain7/1 -> Integrator1/1, wd_ref/1
  Gain9/1 -> ud_ref/1, Integrator3/1
  v_cmd/1 -> Sum1/1
  Sum11/1 -> Gain7/1
  Integrator3/1 -> Sum20/2, u_ref/1
  Sum20/1 -> Gain9/1
  u_cmd/1 -> Sum20/1
  w_cmd/1 -> Sum11/1
  Integrator5/1 -> Sum1/2, v_ref/1
  Gain1/1 -> vd_ref/1, Integrator5/1
  Sum1/1 -> Gain1/1

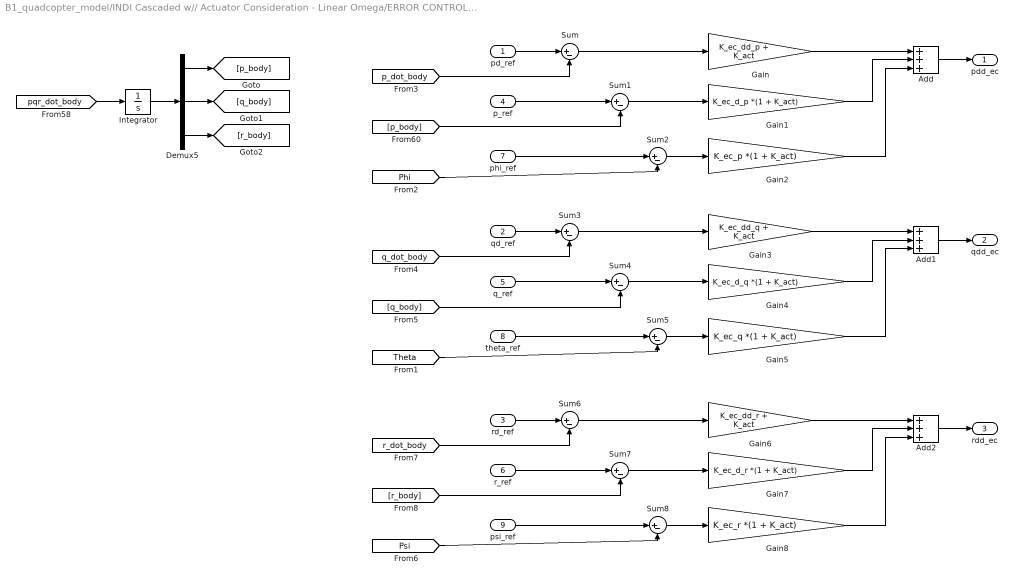
== system B1_quadcopter_model/INDI Cascaded w// Actuator Consideration - Linear Omega/ERROR CONTROLLER ATTITUDE ==
  pd_ref : Inport
  qd_ref : Inport  Port=2
  rd_ref : Inport  Port=3
  p_ref : Inport  Port=4
  q_ref : Inport  Port=5
  r_ref : Inport  Port=6
  phi_ref : Inport  Port=7
  theta_ref : Inport  Port=8
  psi_ref : Inport  Port=9
  Add : Sum  Inputs=+++
  Add1 : Sum  Inputs=+++
  Add2 : Sum  Inputs=+++
  Demux5 : Demux  Outputs=3
  Gain : Gain  Gain=K_ec_dd_p + K_act
  Gain1 : Gain  Gain=K_ec_d_p *(1 + K_act)
  Gain2 : Gain  Gain=K_ec_p *(1 + K_act)
  Gain3 : Gain  Gain=K_ec_dd_q + K_act
  Gain4 : Gain  Gain=K_ec_d_q *(1 + K_act)
  Gain5 : Gain  Gain=K_ec_q *(1 + K_act)
  Gain6 : Gain  Gain=K_ec_dd_r + K_act
  Gain7 : Gain  Gain=K_ec_d_r *(1 + K_act)
  Gain8 : Gain  Gain=K_ec_r *(1 + K_act)
  Integrator : Integrator
  Sum{,1..8} (9 alike) : Sum  Inputs=|+-
  pdd_ec : Outport
  qdd_ec : Outport  Port=2
  rdd_ec : Outport  Port=3
  wires:
  pd_ref/1 -> Sum/1
  p_ref/1 -> Sum1/1
  Add/1 -> pdd_ec/1
  [p_body] -> Sum1/2
  [pqr_dot_body] -> Integrator/1
  Integrator/1 -> Demux5/1
  [Phi] -> Sum2/2
  phi_ref/1 -> Sum2/1
  Demux5/2 -> [q_body]
  Demux5/1 -> [p_body]
  Demux5/3 -> [r_body]
  [p_dot_body] -> Sum/2
  Sum/1 -> Gain/1
  Gain/1 -> Add/1
  Sum1/1 -> Gain1/1
  Sum2/1 -> Gain2/1
  Gain1/1 -> Add/2
  Gain2/1 -> Add/3
  Sum4/1 -> Gain4/1
  Sum5/1 -> Gain5/1
  Sum3/1 -> Gain3/1
  [q_dot_body] -> Sum3/2
  Gain4/1 -> Add1/2
  Gain5/1 -> Add1/3
  theta_ref/1 -> Sum5/1
  [Theta] -> Sum5/2
  [q_body] -> Sum4/2
  Gain3/1 -> Add1/1
  q_ref/1 -> Sum4/1
  Add1/1 -> qdd_ec/1
  qd_ref/1 -> Sum3/1
  Sum7/1 -> Gain7/1
  Sum8/1 -> Gain8/1
  Sum6/1 -> Gain6/1
  [r_dot_body] -> Sum6/2
  Gain7/1 -> Add2/2
  Gain8/1 -> Add2/3
  psi_ref/1 -> Sum8/1
  [Psi] -> Sum8/2
  [r_body] -> Sum7/2
  Gain6/1 -> Add2/1
  r_ref/1 -> Sum7/1
  Add2/1 -> rdd_ec/1
  rd_ref/1 -> Sum6/1

== system B1_quadcopter_model/INDI Cascaded w// Actuator Consideration - Linear Omega/ERROR CONTROLLER VELOCITY ==
  u_ref : Inport
  v_ref : Inport  Port=2
  w_ref : Inport  Port=3
  Gain{,1..5} (6 alike) : Gain  Gain=5
  Integrator : Integrator
  Integrator1 : Integrator
  Integrator2 : Integrator
  Sum : Sum  Inputs=|+-
  Sum1 : Sum  Inputs=|++
  Sum2 : Sum  Inputs=|++
  Sum3 : Sum  Inputs=|+-
  Sum4 : Sum  Inputs=|++
  Sum6 : Sum  Inputs=|+-
  ud_ec : Outport
  vd_ec : Outport  Port=2
  wd_ec : Outport  Port=3
  wires:
  [Vz_earth] -> Sum6/2
  Gain3/1 -> Sum2/2
  Gain1/1 -> Sum1/2
  Sum1/1 -> ud_ec/1
  Gain2/1 -> Sum2/1
  Integrator2/1 -> Gain5/1
  Sum2/1 -> vd_ec/1
  v_ref/1 -> Sum3/1
  Gain4/1 -> Sum4/1
  Integrator1/1 -> Gain3/1
  Gain/1 -> Sum1/1
  u_ref/1 -> Sum/1
  Sum6/1 -> Integrator2/1, Gain4/1
  [Vy_earth] -> Sum3/2
  w_ref/1 -> Sum6/1
  Sum/1 -> Integrator/1, Gain/1
  Sum4/1 -> wd_ec/1
  Gain5/1 -> Sum4/2
  [Vx_earth] -> Sum/2
  Sum3/1 -> Integrator1/1, Gain2/1
  Integrator/1 -> Gain1/1

== system B1_quadcopter_model/INDI Cascaded w// Actuator Consideration - Linear Omega/INTERNAL REFERENCE MODEL ATTITUDE ==
  phi_cmd : Inport
  theta_cmd : Inport  Port=2
  psi_cmd : Inport  Port=3
  Gain1 : Gain  Gain=K_q_dd
  Gain2 : Gain  Gain=K_p_dd
  Gain3 : Gain  Gain=K_r_dd
  Gain4 : Gain  Gain=K_p_d
  Gain5 : Gain  Gain=K_q_d
  Gain6 : Gain  Gain=K_r_d
  Gain7 : Gain  Gain=K_p
  Gain8 : Gain  Gain=K_q
  Gain9 : Gain  Gain=K_r
  Integrator{,1..8} (9 alike) : Integrator
  Subsystem : Subsystem
  Subsystem1 : Subsystem
  Sum{1..4,11,16,20..22} (9 alike) : Sum  Inputs=|+-
  pdd_ref : Outport
  qdd_ref : Outport  Port=2
  rdd_ref : Outport  Port=3
  pd_ref : Outport  Port=4
  qd_ref : Outport  Port=5
  rd_ref : Outport  Port=6
  p_ref : Outport  Port=7
  q_ref : Outport  Port=8
  r_ref : Outport  Port=9
  phi_ref : Outport  Port=10
  theta_ref : Outport  Port=11
  psi_ref : Outport  Port=12
  wires:
  Integrator1/1 -> theta_ref/1, Sum11/2
  Integrator2/1 -> p_ref/1, Subsystem1/1(p), Sum21/2
  Integrator8/1 -> Sum4/2, rd_ref/1, Integrator4/1
  Subsystem1/1(dphi) -> Integrator3/1
  Subsystem1/3(dpsi) -> Integrator5/1
  Subsystem1/2(dtheta) -> Integrator1/1
  Subsystem/2(q) -> Sum16/1
  Subsystem/1(p) -> Sum21/1
  Subsystem/3(r) -> Sum22/1
  Integrator7/1 -> Sum3/2, qd_ref/1, Integrator/1
  Sum21/1 -> Gain4/1
  Sum11/1 -> Gain8/1
  Sum22/1 -> Gain6/1
  Sum16/1 -> Gain5/1
  Integrator3/1 -> phi_ref/1, Sum20/2
  Sum20/1 -> Gain7/1
  Integrator4/1 -> r_ref/1, Subsystem1/3(r), Sum22/2
  Integrator6/1 -> Sum2/2, pd_ref/1, Integrator2/1
  Integrator/1 -> q_ref/1, Subsystem1/2(q), Sum16/2
  phi_cmd/1 -> Sum20/1
  theta_cmd/1 -> Sum11/1
  psi_cmd/1 -> Sum1/1
  Integrator5/1 -> psi_ref/1, Sum1/2
  Sum1/1 -> Gain9/1
  Gain7/1 -> Subsystem/1(dphi)
  Gain8/1 -> Subsystem/2(dtheta)
  Gain9/1 -> Subsystem/3(dpsi)
  Gain4/1 -> Sum2/1
  Gain5/1 -> Sum3/1
  Gain6/1 -> Sum4/1
  Sum2/1 -> Gain2/1
  Sum3/1 -> Gain1/1
  Sum4/1 -> Gain3/1
  Gain2/1 -> pdd_ref/1, Integrator6/1
  Gain1/1 -> qdd_ref/1, Integrator7/1
  Gain3/1 -> rdd_ref/1, Integrator8/1

== system B1_quadcopter_model/INDI Cascaded w// Actuator Consideration - Linear Omega/INTERNAL REFERENCE MODEL VELOCITY ==
  u_cmd : Inport
  v_cmd : Inport  Port=2
  w_cmd : Inport  Port=3
  Gain1 : Gain  Gain=2
  Gain7 : Gain  Gain=2
  Gain9 : Gain  Gain=2
  Integrator1 : Integrator
  Integrator3 : Integrator
  Integrator5 : Integrator
  Sum1 : Sum  Inputs=|+-
  Sum11 : Sum  Inputs=|+-
  Sum20 : Sum  Inputs=|+-
  ud_ref : Outport
  vd_ref : Outport  Port=2
  wd_ref : Outport  Port=3
  u_ref : Outport  Port=4
  v_ref : Outport  Port=5
  w_ref : Outport  Port=6
  wires:
  Integrator1/1 -> w_ref/1, Sum11/2
  Gain7/1 -> Integrator1/1, wd_ref/1
  Gain9/1 -> ud_ref/1, Integrator3/1
  v_cmd/1 -> Sum1/1
  Sum11/1 -> Gain7/1
  Integrator3/1 -> Sum20/2, u_ref/1
  Sum20/1 -> Gain9/1
  u_cmd/1 -> Sum20/1
  w_cmd/1 -> Sum11/1
  Integrator5/1 -> Sum1/2, v_ref/1
  Gain1/1 -> vd_ref/1, Integrator5/1
  Sum1/1 -> Gain1/1

== system B1_quadcopter_model/INDI Cascaded w// State Compensation on qdd/ERROR CONTROLLER ATTITUDE ==
  pd_ref : Inport
  qd_ref : Inport  Port=2
  rd_ref : Inport  Port=3
  p_ref : Inport  Port=4
  q_ref : Inport  Port=5
  r_ref : Inport  Port=6
  phi_ref : Inport  Port=7
  theta_ref : Inport  Port=8
  psi_ref : Inport  Port=9
  Add : Sum  Inputs=+++
  Add1 : Sum  Inputs=+++
  Add2 : Sum  Inputs=+++
  Demux5 : Demux  Outputs=3
  Gain : Gain  Gain=K_ec_dd_p + K_act
  Gain1 : Gain  Gain=K_ec_d_p *(1 + K_act)
  Gain2 : Gain  Gain=K_ec_p *(1 + K_act)
  Gain3 : Gain  Gain=K_ec_dd_q + K_act
  Gain4 : Gain  Gain=K_ec_d_q *(1 + K_act)
  Gain5 : Gain  Gain=K_ec_q *(1 + K_act)
  Gain6 : Gain  Gain=K_ec_dd_r + K_act
  Gain7 : Gain  Gain=K_ec_d_r *(1 + K_act)
  Gain8 : Gain  Gain=K_ec_r *(1 + K_act)
  Integrator : Integrator
  Sum{,1..8} (9 alike) : Sum  Inputs=|+-
  pdd_ec : Outport
  qdd_ec : Outport  Port=2
  rdd_ec : Outport  Port=3
  wires:
  pd_ref/1 -> Sum/1
  p_ref/1 -> Sum1/1
  Add/1 -> pdd_ec/1
  [p_body] -> Sum1/2
  [pqr_dot_body] -> Integrator/1
  Integrator/1 -> Demux5/1
  [Phi] -> Sum2/2
  phi_ref/1 -> Sum2/1
  Demux5/2 -> [q_body]
  Demux5/1 -> [p_body]
  Demux5/3 -> [r_body]
  [p_dot_body] -> Sum/2
  Sum/1 -> Gain/1
  Gain/1 -> Add/1
  Sum1/1 -> Gain1/1
  Sum2/1 -> Gain2/1
  Gain1/1 -> Add/2
  Gain2/1 -> Add/3
  Sum4/1 -> Gain4/1
  Sum5/1 -> Gain5/1
  Sum3/1 -> Gain3/1
  [q_dot_body] -> Sum3/2
  Gain4/1 -> Add1/2
  Gain5/1 -> Add1/3
  theta_ref/1 -> Sum5/1
  [Theta] -> Sum5/2
  [q_body] -> Sum4/2
  Gain3/1 -> Add1/1
  q_ref/1 -> Sum4/1
  Add1/1 -> qdd_ec/1
  qd_ref/1 -> Sum3/1
  Sum7/1 -> Gain7/1
  Sum8/1 -> Gain8/1
  Sum6/1 -> Gain6/1
  [r_dot_body] -> Sum6/2
  Gain7/1 -> Add2/2
  Gain8/1 -> Add2/3
  psi_ref/1 -> Sum8/1
  [Psi] -> Sum8/2
  [r_body] -> Sum7/2
  Gain6/1 -> Add2/1
  r_ref/1 -> Sum7/1
  Add2/1 -> rdd_ec/1
  rd_ref/1 -> Sum6/1

== system B1_quadcopter_model/INDI Cascaded w// State Compensation on qdd/ERROR CONTROLLER VELOCITY ==
  u_ref : Inport
  v_ref : Inport  Port=2
  w_ref : Inport  Port=3
  Gain{,1..5} (6 alike) : Gain  Gain=5
  Integrator : Integrator
  Integrator1 : Integrator
  Integrator2 : Integrator
  Sum : Sum  Inputs=|+-
  Sum1 : Sum  Inputs=|++
  Sum2 : Sum  Inputs=|++
  Sum3 : Sum  Inputs=|+-
  Sum4 : Sum  Inputs=|++
  Sum6 : Sum  Inputs=|+-
  ud_ec : Outport
  vd_ec : Outport  Port=2
  wd_ec : Outport  Port=3
  wires:
  [Vz_earth] -> Sum6/2
  Gain3/1 -> Sum2/2
  Gain1/1 -> Sum1/2
  Sum1/1 -> ud_ec/1
  Gain2/1 -> Sum2/1
  Integrator2/1 -> Gain5/1
  Sum2/1 -> vd_ec/1
  v_ref/1 -> Sum3/1
  Gain4/1 -> Sum4/1
  Integrator1/1 -> Gain3/1
  Gain/1 -> Sum1/1
  u_ref/1 -> Sum/1
  Sum6/1 -> Integrator2/1, Gain4/1
  [Vy_earth] -> Sum3/2
  w_ref/1 -> Sum6/1
  Sum/1 -> Integrator/1, Gain/1
  Sum4/1 -> wd_ec/1
  Gain5/1 -> Sum4/2
  [Vx_earth] -> Sum/2
  Sum3/1 -> Integrator1/1, Gain2/1
  Integrator/1 -> Gain1/1

== system B1_quadcopter_model/INDI Cascaded w// State Compensation on qdd/INTERNAL REFERENCE MODEL ATTITUDE ==
  phi_cmd : Inport
  theta_cmd : Inport  Port=2
  psi_cmd : Inport  Port=3
  Gain1 : Gain  Gain=K_q_dd
  Gain2 : Gain  Gain=K_p_dd
  Gain3 : Gain  Gain=K_r_dd
  Gain4 : Gain  Gain=K_p_d
  Gain5 : Gain  Gain=K_q_d
  Gain6 : Gain  Gain=K_r_d
  Gain7 : Gain  Gain=K_p
  Gain8 : Gain  Gain=K_q
  Gain9 : Gain  Gain=K_r
  Integrator{,1..8} (9 alike) : Integrator
  Subsystem : Subsystem
  Subsystem1 : Subsystem
  Sum{1..4,11,16,20..22} (9 alike) : Sum  Inputs=|+-
  pdd_ref : Outport
  qdd_ref : Outport  Port=2
  rdd_ref : Outport  Port=3
  pd_ref : Outport  Port=4
  qd_ref : Outport  Port=5
  rd_ref : Outport  Port=6
  p_ref : Outport  Port=7
  q_ref : Outport  Port=8
  r_ref : Outport  Port=9
  phi_ref : Outport  Port=10
  theta_ref : Outport  Port=11
  psi_ref : Outport  Port=12
  wires:
  Integrator1/1 -> theta_ref/1, Sum11/2
  Integrator2/1 -> p_ref/1, Subsystem1/1(p), Sum21/2
  Integrator8/1 -> Sum4/2, rd_ref/1, Integrator4/1
  Subsystem1/1(dphi) -> Integrator3/1
  Subsystem1/3(dpsi) -> Integrator5/1
  Subsystem1/2(dtheta) -> Integrator1/1
  Subsystem/2(q) -> Sum16/1
  Subsystem/1(p) -> Sum21/1
  Subsystem/3(r) -> Sum22/1
  Integrator7/1 -> Sum3/2, qd_ref/1, Integrator/1
  Sum21/1 -> Gain4/1
  Sum11/1 -> Gain8/1
  Sum22/1 -> Gain6/1
  Sum16/1 -> Gain5/1
  Integrator3/1 -> phi_ref/1, Sum20/2
  Sum20/1 -> Gain7/1
  Integrator4/1 -> r_ref/1, Subsystem1/3(r), Sum22/2
  Integrator6/1 -> Sum2/2, pd_ref/1, Integrator2/1
  Integrator/1 -> q_ref/1, Subsystem1/2(q), Sum16/2
  phi_cmd/1 -> Sum20/1
  theta_cmd/1 -> Sum11/1
  psi_cmd/1 -> Sum1/1
  Integrator5/1 -> psi_ref/1, Sum1/2
  Sum1/1 -> Gain9/1
  Gain7/1 -> Subsystem/1(dphi)
  Gain8/1 -> Subsystem/2(dtheta)
  Gain9/1 -> Subsystem/3(dpsi)
  Gain4/1 -> Sum2/1
  Gain5/1 -> Sum3/1
  Gain6/1 -> Sum4/1
  Sum2/1 -> Gain2/1
  Sum3/1 -> Gain1/1
  Sum4/1 -> Gain3/1
  Gain2/1 -> pdd_ref/1, Integrator6/1
  Gain1/1 -> qdd_ref/1, Integrator7/1
  Gain3/1 -> rdd_ref/1, Integrator8/1

== system B1_quadcopter_model/INDI Cascaded w// State Compensation on qdd/INTERNAL REFERENCE MODEL VELOCITY ==
  u_cmd : Inport
  v_cmd : Inport  Port=2
  w_cmd : Inport  Port=3
  Gain1 : Gain  Gain=2
  Gain7 : Gain  Gain=2
  Gain9 : Gain  Gain=2
  Integrator1 : Integrator
  Integrator3 : Integrator
  Integrator5 : Integrator
  Sum1 : Sum  Inputs=|+-
  Sum11 : Sum  Inputs=|+-
  Sum20 : Sum  Inputs=|+-
  ud_ref : Outport
  vd_ref : Outport  Port=2
  wd_ref : Outport  Port=3
  u_ref : Outport  Port=4
  v_ref : Outport  Port=5
  w_ref : Outport  Port=6
  wires:
  Integrator1/1 -> w_ref/1, Sum11/2
  Gain7/1 -> Integrator1/1, wd_ref/1
  Gain9/1 -> ud_ref/1, Integrator3/1
  v_cmd/1 -> Sum1/1
  Sum11/1 -> Gain7/1
  Integrator3/1 -> Sum20/2, u_ref/1
  Sum20/1 -> Gain9/1
  u_cmd/1 -> Sum20/1
  w_cmd/1 -> Sum11/1
  Integrator5/1 -> Sum1/2, v_ref/1
  Gain1/1 -> vd_ref/1, Integrator5/1
  Sum1/1 -> Gain1/1

== system B1_quadcopter_model/INDI Cascaded w// State Compensation on qdd/STATE COMPENSATION BLOCK ==
  Derivative{,1..3} (4 alike) : Derivative
  Manual Switch : ManualSwitch  CurrentSetting=0
  Manual Switch1 : ManualSwitch  CurrentSetting=0
  Manual Switch2 : ManualSwitch
  Mathematical Derivation : MATLAB Function  TreatAsAtomicUnit=on
  Moment Block form Plant - Plant States : Subsystem
  "Moment Block form Plant - Reference States " : Subsystem
  Straight up formula + derivative : MATLAB Function  TreatAsAtomicUnit=on
  qdd_x : Outport
  wires:
  [Vx_body] -> Mathematical Derivation/5(u_b)
  [Iyy] -> Straight up formula + derivative/3(Iyy)
  [r_plate] -> Straight up formula + derivative/1(r_plate)
  Straight up formula + derivative/1(qd_x) -> Derivative1/1
  [Ax_body] -> Mathematical Derivation/9(ud_b)
  [Ay_body] -> Mathematical Derivation/10(vd_b)
  [Az_body] -> Mathematical Derivation/11(wd_b)
  [r_plate] -> Mathematical Derivation/1(r_plate)
  [l_plate] -> Mathematical Derivation/2(l_plate)
  [l_plate] -> Straight up formula + derivative/2(l_plate)
  [rho] -> Straight up formula + derivative/4(rho)
  [Vy_body] -> Straight up formula + derivative/6(v_b)
  [Iyy] -> Mathematical Derivation/3(Iyy)
  [Vx_body] -> Straight up formula + derivative/5(u_b)
  [Vz_body] -> Straight up formula + derivative/7(w_b)
  [rho] -> Mathematical Derivation/4(rho)
  [alpha] -> Derivative/1, Mathematical Derivation/8(alpha)
  [Vy_body] -> Mathematical Derivation/6(v_b)
  [alpha] -> Straight up formula + derivative/8(alpha)
  Derivative/1 -> Mathematical Derivation/12(alphad)
  [Vz_body] -> Mathematical Derivation/7(w_b)
  Mathematical Derivation/1(qdd_x) -> Manual Switch/1
  Manual Switch/1 -> qdd_x/1
  Moment Block form Plant - Plant States/1(qd) -> Derivative2/1
  Manual Switch1/1 -> Manual Switch/2
  Derivative1/1 -> Manual Switch1/1
  "Moment Block form Plant - Reference States "/1(qd) -> Derivative3/1
  Manual Switch2/1 -> Manual Switch1/2
  Derivative2/1 -> Manual Switch2/1
  Derivative3/1 -> Manual Switch2/2
